simulink model "L4_MABX"  (R2018a)
settings: Solver=FixedStepDiscrete  StartTime=0.0  StopTime=Inf  FixedStep=0.01  RelTol=1e-3  EnableMultiTasking=on
PostLoadFcn:
  | , if any(exist('dsrtsu_mdlpostloadfcn', 'file') == [2, 3, 6]), try dsrtsu_mdlpostloadfcn('Execute', bdroot); catch fprintf('Error in PostLoadFcn (dsrtsu_mdlpostloadfcn) for model "%s":\n %s\n', bdroot, lasterr); end, end,
InitFcn:
  | disp([ptc_matlab_lib.isodatetime ' - ' bdroot(gcs) ' - Setting FixedStep to GLB_FIXED_STEP_SIZE_CPV']);
  | set_param(bdroot(gcs), 'FixedStep', num2str(GLB_FIXED_STEP_SIZE_CPV.Value));
undefined symbols (not defined in the file or in its folder): dsa_RTMapsManager, ENUM_CAN_STATUS_DIAG_T
libraries: PTC_MBDS_LIB x14, rtican x12, dsa_tcpip_lib x2, SUB_ECU_L4_MABX_HW_Interface_PIC_KW x2, rtiethxcplib x2, SUB_ECU_L4_MABX x1, simulink x1, rtmapslib x1
(part 1 of 2)
settings Model: DSRTSU_INTERNAL_RTI_VER=520  DSRTSU_INTERNAL_RTI_TYPE=rti1401  DSRTSU_INTERNAL_RTIFPGA=110  RTICANMMDATA=struct('GeneralSetupData',struct('modelroot','C:\Users\Gavin.Coelho\Repos\mabx\src','generalsettings',struct('filesettings',struct('destfolder',struct('Name','RTICANMM_FILES','Check',1),'buildfolder',struct('Name','.','Check',1),'AbsDestfolder',struct('Name','C:\Users\Gavin.Coelho\Repos\mabx\src\RTICANMM_FILES'),'AbsBuildfolder',struct('Name','C:\Users\Gavin.Coelho\Repos\mabx\src'))),'options',struct('addpaths',1,'rmpaths',1,'addtrcexclusion',logical(1),'cannavigator',struct('checkmonitoring',0),'show_usrtrc',0,'use_usrtrc',0),'advanced',struct('options',[1 1 1 1 1 1 1 1 1 1 1 1 1 1 1 1 1 1 1 1 1 1 1 1 1 1 1 1 1 1 1 1 1 1 1 1 1 1 1 1 1 1 1 1 1 1 1 1 1 1 1 1 1 1 1 1 1 1 1 1 1 1 1 1 1 1 1 1 1 1 1 1 1 1 1 1 1 1 1 1 1 1 1 1 1 1 1 1 1 1 1 1 1 1 1 1 1 1 1 1]),'MPSetup',{{}},'modelname','L4_MABX','block','L4_MABX'))  DSRTSU_INTERNAL_RTIFLEXRAYCONFIG=110  Creator=charles.swart  LastModifiedBy=Gavin.Coelho
settings SolverCC: AutoInsertRateTranBlk=on  InsertRTBMode=Always
settings DataIOCC: LimitDataPoints=on  SaveFormat=Array
settings OptimizationCC: BlockReduction=off  OptimizeBlockIOStorage=off  BufferReuse=off  GlobalBufferReuse=off  ExpressionFolding=off  LocalBlockOutputs=off  LifeSpan=inf  OptimizeDataStoreBuffers=off  BusAssignmentInplaceUpdate=off
settings DebuggingCC: SolverPrmCheckMsg=warning  MultiTaskDSMMsg=warning  MultiTaskCondExecSysMsg=warning  MultiTaskRateTransMsg=warning  ParameterPrecisionLossMsg=none  SignalLabelMismatchMsg=warning  UnconnectedInputMsg=error  UnconnectedLineMsg=error  StrictBusMsg=WarnOnBusTreatedAsVector  NonBusSignalsTreatedAsBus=warning  SFUnexpectedBacktrackingDiag=warning  SFNoUnconditionalDefaultTransitionDiag=warning  SFExecutionAtInitializationDiag=none
settings HardwareCC: ProdBitPerPointer=32  ProdBitPerSizeT=32  ProdBitPerPtrDiffT=32  ProdLargestAtomicInteger=Integer  ProdEndianess=BigEndian  ProdWordSize=32  ProdHWDeviceType=Custom Processor->Custom  TargetIntDivRoundTo=Zero  TargetEndianess=BigEndian  TargetHWDeviceType=Custom Processor->Custom
settings ModelReferenceCC: PropagateSignalLabelsOutOfModel=off
settings SFSimCC: MATLABDynamicMemAlloc=off
settings RTWCC: SystemTargetFile=rti1401.tlc  MakeCommand=make_rti  TemplateMakefile=rti1401.tmf  Description=dSPACE DS1401 Hardware Platform  GenerateReport=on
settings CodeAppCC: StateflowObjectComments=on
settings STFCustomTargetCC: ParMdlRefBuildCompliant=on  GRTInterface=off  SystemTargetFile=rti1401.tlc
settings GRTTargetCC: TargetLangStandard=C89/C90 (ANSI)  CompOptLevelCompliant=off  ConcurrentExecutionCompliant=off  CombineOutputUpdateFcns=off  MatFileLogging=off  CPPClassGenCompliant=off  UseToolchainInfoCompliant=off  ExtModeMexFile=noextcomm
settings ConfigComp: CovMetricSettings=dw  CovHtmlReporting=on  CovSaveCumulativeToWorkspaceVar=on  CovSaveSingleToWorkspaceVar=on  CovExternalEMLEnable=off  CovSFcnEnable=off

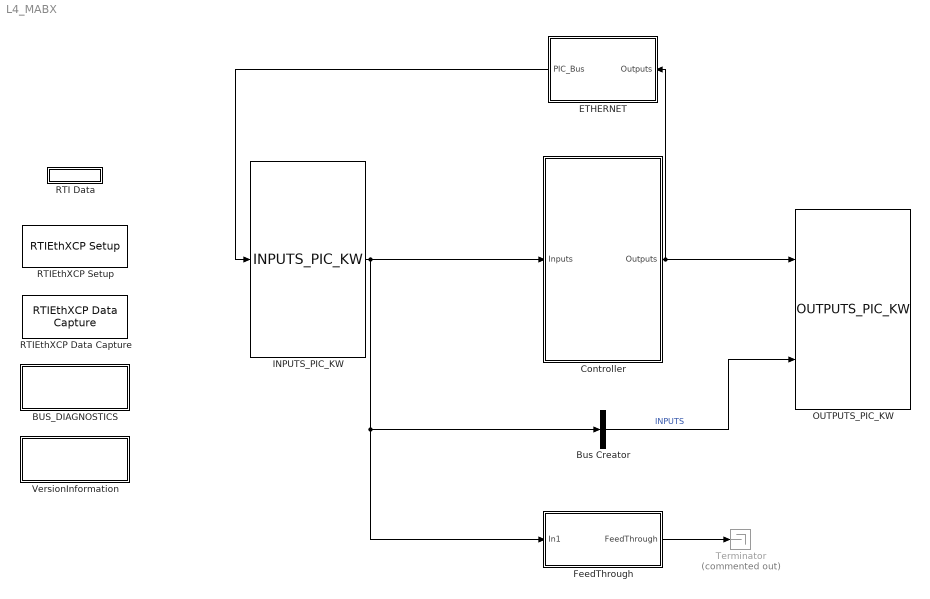
== system L4_MABX ==
  BUS_DIAGNOSTICS : Subsystem
  Bus Creator : BusCreator  Inputs=1
  Controller : Subsystem
  ETHERNET : Subsystem  AncestorBlock=SUB_ECU_L4_MABX_HW_Interface_PIC_KW/ETHERNET
  FeedThrough : Subsystem
  INPUTS_PIC_KW : SUB_ECU_L4_MABX_HW_Interface_PIC_KW/INPUTS_PIC_KW
      link override DIGITAL/Constant2: Value=1000
  OUTPUTS_PIC_KW : SUB_ECU_L4_MABX_HW_Interface_PIC_KW/OUTPUTS_PIC_KW
  RTI Data : Subsystem  Tag=struct('RTIDataServer',struct('RTIDataServerVs','2','RTIModelDescription','struct(''main'',''L4_MABX'',''sub'','''',''isMp'',0)'))  LoadFcn="if exist('rtidc'), try,  rtidc('DataHostBlockClbLoad', gcbh); catch, disp(['Warning: ''LoadFcn'' for RTI Data block failed: ' lasterr]); end, end,"  mask(RTI_DATA_HOST){}
      mask help:
      | RTI Data Block.
      | This block is used by RTI to store internal model-dependent data.
      | Please keep this block on the root level of the model. Deleting this block will result in data loss.
      |
      | NEVER DELETE OR COPY THIS BLOCK!
      settings: CopyFcn="if exist('rtidc'), try,  rtidc('DataHostBlockClbCopy', gcbh); catch, disp(['Warning: ''CopyFcn'' for RTI Data block failed: ' lasterr]); end, end,"  DeleteFcn="if exist('rtidc'), try,  rtidc('DataHostBlockClbDelete', gcbh); catch, disp(['Warning: ''DeleteFcn'' for RTI Data block failed: ' lasterr]); end, end,"  ModelCloseFcn="if exist('rtidc'), try,  rtidc('DataHostBlockClbModelClose', gcbh); catch, disp(['Warning: ''ModelCloseFcn'' for RTI Data block failed: ' lasterr]); end, end,"  PreSaveFcn="if exist('rtidc'), try,  rtidc('DataHostBlockClbPreSave', gcbh); catch, disp(['Warning: ''PreSaveFcn'' for RTI Data block failed: ' lasterr]); end, end,"  PostSaveFcn="if exist('rtidc'), try,  rtidc('DataHostBlockClbPostSave', gcbh); catch, disp(['Warning: ''PostSaveFcn'' for RTI Data block failed: ' lasterr]); end, end,"  NameChangeFcn="if exist('rtidc'), try,  rtidc('DataHostBlockClbNameChange', gcbh); catch, disp(['Warning: ''NameChangeFcn'' for RTI Data block failed: ' lasterr]); end, end,"
      mask Help:
      | RTI Data Block.
      | This block is used by RTI to store internal model-dependent data.
      | Please keep this block on the root level of the model. Deleting this block will result in data loss.
      | 
      | NEVER DELETE OR COPY THIS BLOCK!
      mask Display:
      | text(0.5, 0.5, 'RTI Data', 'HorizontalAlignment', 'center');
      | plot([1 0]);
  RTIEthXCP Data Capture : rtiethxcplib/RTIEthXCP Data Capture  Reserved1=[]  Reserved2=[]  Reserved3=[]  Reserved4=[]  DSProperties=struct('RTI',struct('Version',uint32(1),'BlockType',struct('isSLSource',uint8(0),'isSLSink',uint8(0),'isHWSource',uint8(0),'isHWSink',uint8(0),'isSetup',uint8(0),'isInline',uint8(1),'isNonInline',uint8(0),'isInterrupt',uint8(0),'isChannelwise',uint8(0)),'IOBoardType','RTIETHXCP','UnitType','NON_MESSAGE','Identifier','DATACAPTURE','DialogType','ML','BlockSet','RTIETHXCP','SlaveProcessor','NONE'))  RTIBlockInterface=struct('DialogFcn','guiethxcpdatacapture','BlockDisplay',{{['XCP Service #0\n<event channel name>\nCapture at task: <end>'],'center'}},'OutputPortsWidth',int32(0),'OutputPortsActive',0,'IconTransparency','on','InitLevel',3,'SampleTime',{{-1}},'BlockName',struct('Token',{{['RTIEthXCP Data Capture']}}))  RTIBlockParameters=struct('EventChannelName',{{'event_channel','OFF',[]}},'EventChannelNumber',{{0,'OFF',[]}},'DataCaptureAtEnd',{{1,'OFF',[0 1]}},'NumFormat',{{'dec','OFF',[]}},'SampleTime',{{-1,'OFF',[]}},'blockParam',{{0,'OFF',[]}},'TLCFileName',{{'rtiethxcpdatacapture','OFF',[]}})  RTISFcnParameters=struct('blockParam','struct','TLCFileName','char')  RTIBlockParaDefault=struct('EventChannelName','event_channel','EventChannelNumber',0,'DataCaptureAtEnd',1,'NumFormat','dec','SampleTime',-1,'blockParam',0,'TLCFileName','rtiethxcpdatacapture')
      settings: SourceProductName=dSPACE RTI XCP on Ethernet Blockset
  RTIEthXCP Setup : rtiethxcplib/RTIEthXCP Setup  Reserved1=[]  Reserved2=[]  Reserved3=[]  Reserved4=[]  DSProperties=struct('RTI',struct('Version',uint32(1),'BlockType',struct('isSLSource',uint8(0),'isSLSink',uint8(0),'isHWSource',uint8(0),'isHWSink',uint8(0),'isSetup',uint8(0),'isInline',uint8(1),'isNonInline',uint8(0),'isInterrupt',uint8(0),'isChannelwise',uint8(0)),'IOBoardType','RTIETHXCP','UnitType','NON_MESSAGE','Identifier','SETUP','DialogType','ML','BlockSet','RTIETHXCP','SlaveProcessor','NONE'))  RTIBlockInterface=struct('DialogFcn','guiethxcpsetup','BlockDisplay',{{['RTI Ethernet XCP\nSETUP'],'center'}},'OutputPortsWidth',int32(0),'OutputPortsActive',0,'IconTransparency','on','InitLevel',3,'SampleTime',{{-1}},'BlockName',struct('Token',{{['RTIEthXCP Setup']}}))  RTIBlockParameters=struct('BoardNo',{{1,'ON',[1 16]}},'UseStaticDAQLists',{{0,'OFF',[0 1]}},'Port',{{1234,'ON',[1 65535]}},'EthernetInterface',{{1,'OFF',[0 1]}},'blockParam',{{0,'OFF',[]}},'TLCFileName',{{'rtiethxcpsetup','OFF',[]}},'Address',{{'192.168.140.1','OFF',[]}},'VECUStruct',{{struct('EnableVECUA2LMerging',0,'SrcA2LFileName','','EVENTs',[]),'OFF',[]}})  RTISFcnParameters=struct('blockParam','struct','TLCFileName','char')  RTIBlockParaDefault=struct('BoardNo',1,'UseStaticDAQLists',0,'Port',1234,'EthernetInterface',0,'blockParam',0,'TLCFileName','rtiethxcpsetup','Address','127.0.0.1','VECUStruct',struct('EnableVECUA2LMerging',0,'SrcA2LFileName','','EVENTs',[]))
      settings: SourceProductName=dSPACE RTI XCP on Ethernet Blockset
  Terminator : Terminator  Commented=on
      settings: InitFcn=|
      | try
      |    MBDS_BlockCallback('Update', gcb);
      | end
  VersionInformation : Subsystem
  wires:
  FeedThrough/1(FeedThrough) -> Terminator/1
  INPUTS_PIC_KW/1 -> Bus Creator/1, FeedThrough/1(In1), Controller/1(Inputs)
  Controller/1(Outputs) -> OUTPUTS_PIC_KW/1, ETHERNET/1(Outputs)
  Bus Creator/1 -> OUTPUTS_PIC_KW/2  "INPUTS"
  ETHERNET/1(PIC_Bus) -> INPUTS_PIC_KW/1

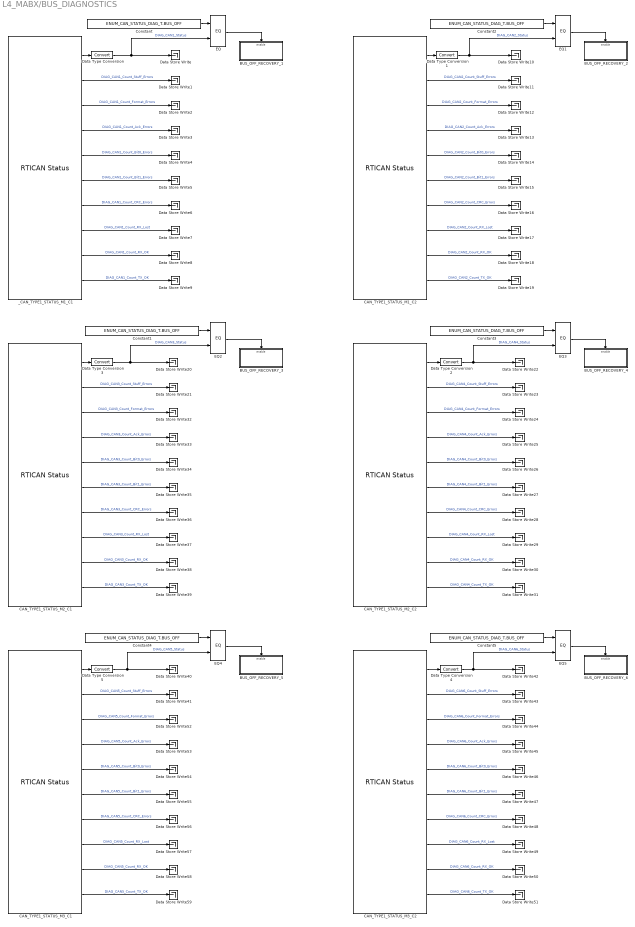
== system L4_MABX/BUS_DIAGNOSTICS ==
  BUS_OFF_RECOVERY_1 : Subsystem
  BUS_OFF_RECOVERY_2 : Subsystem
  BUS_OFF_RECOVERY_3 : Subsystem
  BUS_OFF_RECOVERY_4 : Subsystem
  BUS_OFF_RECOVERY_5 : Subsystem
  BUS_OFF_RECOVERY_6 : Subsystem
  CAN_TYPE1_STATUS_M1_C2 : rtican/RTICAN Status   Reserved1=[]  Reserved2=[]  Reserved3=[]  Reserved4=[]  DialogFcn=[]  UnitName=[]  SFcnRTICANStatus=[]  BoardTypeNo=[]  BoardNo=[]  ChannelNo=[]  Parameters=[]  Revision=[]  UnitValues=[]  DSProperties=struct('RTI',struct('Version',uint32(4),'BlockType',struct('isSLSource',uint8(1),'isSLSink',uint8(0),'isHWSource',uint8(0),'isHWSink',uint8(0),'isSetup',uint8(0),'isInline',uint8(1),'isNonInline',uint8(0),'isInterrupt',uint8(0),'isChannelwise',uint8(0)),'IOBoardType','RTICAN','UnitType','NON_MESSAGE','Identifier','STATUS','DialogType','ML','BlockSet','RTICAN','SlaveProcessor','CAN'))  RTIBlockInterface=struct('OutputPortsWidth',int32([1 1 1 1 1 1 1 1 1 1 1 1]),'OutputPortsActive',[1 1 1 1 1 1 1 1 1 1 0 0],'OutputPortsName',{{'Status',['Stuff errors'],['Format errors'],['Ack errors'],['Bit 0 errors'],['Bit 1 errors'],['CRC errors'],['RX lost'],['RX ok'],['TX ok'],['FT Status'],['FT error count']}},'OutputPortsDataType',{{'SS_UINT32','SS_UINT32','SS_UINT32','SS_UINT32','SS_UINT32','SS_UINT32','SS_UINT32','SS_UINT32','SS_UINT32','SS_UINT32','SS_UINT32','SS_UINT32'}},'DialogFcn','rtican_status_gui','BlockDisplay',{{'','center'}},'IconTransparency','on','ParameterTunableNames',{{}},'InitLevel',3,'BlockName',struct('Token',{{'CAN_TYPE','_STATUS_M','_C'}},'BlockParam',{{'BoardTypeNo','BoardNo','ChannelNo'}}),'SampleTime',{{2^-1}})  RTIBlockParameters=struct('BoardTypeNo',{{1,'OFF',[]}},'BoardNo',{{1,'ON',[1 16]}},'ChannelNo',{{2,'ON',[1 2]}},'Parameters',{{struct('general',struct('isFromLib',0,'StatusFlags',{{1;1;1;1;1;1;1;1;1;1;0;0}}),'options',struct('SampleTime',2^-1)),'OFF',[]}},'GroupId',{{struct('Group','RTICAN','No',2,'Behavior','NAMECHANGE','BlockType','SINK','NameChangeFlag',0),'OFF',[]}},'SFcnRTICANStatus',{{struct('Output',struct('Name',{'Status','StuffErrors','FormatErrors','AckErrors','Bit0Errors','Bit1Errors','CRCErrors','RXLost','RXOK','TXOK','FTStatus','FTErrorCount'},'Selected',{'yes','yes','yes','yes','yes','yes','yes','yes','yes','yes','no','no'}),'ControllerNo',2,'BoardNo',1,'BoardType','DS1','PortDatatype','UInt32'),'OFF',[]}},'TLCFileName',{{'rtican_status','OFF',[]}})  RTISFcnParameters=struct('SFcnRTICANStatus','struct','TLCFileName','char')  RTIBlockParaDefault=struct('BoardTypeNo',4302,'BoardNo',1,'ChannelNo',1,'Parameters',struct('general',struct('StatusFlags',{{1;1;1;1;1;1;1;1;1;1;0;0}},'isFromLib',1),'options',struct('SampleTime',2^-1)),'GroupId',struct('Group',{{'RTICAN'}},'No',1,'Behavior',{{'NAMECHANGE'}},'BlockType',{{'SINK'}},'NameChangeFlag',0),'SFcnRTICANStatus',struct('Output',struct('Name',{'Status','StuffErrors','FormatErrors','AckErrors','Bit0Errors','Bit1Errors','CRCErrors','RXLost','RXOK','TXOK','FTStatus','FTErrorCount'},'Selected',{'yes','yes','yes','yes','yes','yes','yes','yes','yes','yes','no','no'}),'ControllerNo',1,'BoardNo',1,'BoardType','DS4302','PortDatatype','real_T'),'TLCFileName','rtican_status')
      settings: AttributesFormatString=Group Id: RTICAN2\n  SourceProductName=dSPACE RTI CAN Blockset
  CAN_TYPE1_STATUS_M2_C1 : rtican/RTICAN Status   Reserved1=[]  Reserved2=[]  Reserved3=[]  Reserved4=[]  DialogFcn=[]  UnitName=[]  SFcnRTICANStatus=[]  BoardTypeNo=[]  BoardNo=[]  ChannelNo=[]  Parameters=[]  Revision=[]  UnitValues=[]  DSProperties=struct('RTI',struct('Version',uint32(4),'BlockType',struct('isSLSource',uint8(1),'isSLSink',uint8(0),'isHWSource',uint8(0),'isHWSink',uint8(0),'isSetup',uint8(0),'isInline',uint8(1),'isNonInline',uint8(0),'isInterrupt',uint8(0),'isChannelwise',uint8(0)),'IOBoardType','RTICAN','UnitType','NON_MESSAGE','Identifier','STATUS','DialogType','ML','BlockSet','RTICAN','SlaveProcessor','CAN'))  RTIBlockInterface=struct('OutputPortsWidth',int32([1 1 1 1 1 1 1 1 1 1 1 1]),'OutputPortsActive',[1 1 1 1 1 1 1 1 1 1 0 0],'OutputPortsName',{{'Status',['Stuff errors'],['Format errors'],['Ack errors'],['Bit 0 errors'],['Bit 1 errors'],['CRC errors'],['RX lost'],['RX ok'],['TX ok'],['FT Status'],['FT error count']}},'OutputPortsDataType',{{'SS_UINT32','SS_UINT32','SS_UINT32','SS_UINT32','SS_UINT32','SS_UINT32','SS_UINT32','SS_UINT32','SS_UINT32','SS_UINT32','SS_UINT32','SS_UINT32'}},'DialogFcn','rtican_status_gui','BlockDisplay',{{'','center'}},'IconTransparency','on','ParameterTunableNames',{{}},'InitLevel',3,'BlockName',struct('Token',{{'CAN_TYPE','_STATUS_M','_C'}},'BlockParam',{{'BoardTypeNo','BoardNo','ChannelNo'}}),'SampleTime',{{2^-1}})  RTIBlockParameters=struct('BoardTypeNo',{{1,'OFF',[]}},'BoardNo',{{2,'ON',[1 16]}},'ChannelNo',{{1,'ON',[1 2]}},'Parameters',{{struct('general',struct('isFromLib',0,'StatusFlags',{{1;1;1;1;1;1;1;1;1;1;0;0}}),'options',struct('SampleTime',2^-1)),'OFF',[]}},'GroupId',{{struct('Group','RTICAN','No',3,'Behavior','NAMECHANGE','BlockType','SINK','NameChangeFlag',0),'OFF',[]}},'SFcnRTICANStatus',{{struct('Output',struct('Name',{'Status','StuffErrors','FormatErrors','AckErrors','Bit0Errors','Bit1Errors','CRCErrors','RXLost','RXOK','TXOK','FTStatus','FTErrorCount'},'Selected',{'yes','yes','yes','yes','yes','yes','yes','yes','yes','yes','no','no'}),'ControllerNo',1,'BoardNo',2,'BoardType','DS1','PortDatatype','UInt32'),'OFF',[]}},'TLCFileName',{{'rtican_status','OFF',[]}})  RTISFcnParameters=struct('SFcnRTICANStatus','struct','TLCFileName','char')  RTIBlockParaDefault=struct('BoardTypeNo',4302,'BoardNo',1,'ChannelNo',1,'Parameters',struct('general',struct('StatusFlags',{{1;1;1;1;1;1;1;1;1;1;0;0}},'isFromLib',1),'options',struct('SampleTime',2^-1)),'GroupId',struct('Group',{{'RTICAN'}},'No',1,'Behavior',{{'NAMECHANGE'}},'BlockType',{{'SINK'}},'NameChangeFlag',0),'SFcnRTICANStatus',struct('Output',struct('Name',{'Status','StuffErrors','FormatErrors','AckErrors','Bit0Errors','Bit1Errors','CRCErrors','RXLost','RXOK','TXOK','FTStatus','FTErrorCount'},'Selected',{'yes','yes','yes','yes','yes','yes','yes','yes','yes','yes','no','no'}),'ControllerNo',1,'BoardNo',1,'BoardType','DS4302','PortDatatype','real_T'),'TLCFileName','rtican_status')
      settings: AttributesFormatString=Group Id: RTICAN3\n  SourceProductName=dSPACE RTI CAN Blockset
  CAN_TYPE1_STATUS_M2_C2 : rtican/RTICAN Status   Reserved1=[]  Reserved2=[]  Reserved3=[]  Reserved4=[]  DialogFcn=[]  UnitName=[]  SFcnRTICANStatus=[]  BoardTypeNo=[]  BoardNo=[]  ChannelNo=[]  Parameters=[]  Revision=[]  UnitValues=[]  DSProperties=struct('RTI',struct('Version',uint32(4),'BlockType',struct('isSLSource',uint8(1),'isSLSink',uint8(0),'isHWSource',uint8(0),'isHWSink',uint8(0),'isSetup',uint8(0),'isInline',uint8(1),'isNonInline',uint8(0),'isInterrupt',uint8(0),'isChannelwise',uint8(0)),'IOBoardType','RTICAN','UnitType','NON_MESSAGE','Identifier','STATUS','DialogType','ML','BlockSet','RTICAN','SlaveProcessor','CAN'))  RTIBlockInterface=struct('OutputPortsWidth',int32([1 1 1 1 1 1 1 1 1 1 1 1]),'OutputPortsActive',[1 1 1 1 1 1 1 1 1 1 0 0],'OutputPortsName',{{'Status',['Stuff errors'],['Format errors'],['Ack errors'],['Bit 0 errors'],['Bit 1 errors'],['CRC errors'],['RX lost'],['RX ok'],['TX ok'],['FT Status'],['FT error count']}},'OutputPortsDataType',{{'SS_UINT32','SS_UINT32','SS_UINT32','SS_UINT32','SS_UINT32','SS_UINT32','SS_UINT32','SS_UINT32','SS_UINT32','SS_UINT32','SS_UINT32','SS_UINT32'}},'DialogFcn','rtican_status_gui','BlockDisplay',{{'','center'}},'IconTransparency','on','ParameterTunableNames',{{}},'InitLevel',3,'BlockName',struct('Token',{{'CAN_TYPE','_STATUS_M','_C'}},'BlockParam',{{'BoardTypeNo','BoardNo','ChannelNo'}}),'SampleTime',{{2^-1}})  RTIBlockParameters=struct('BoardTypeNo',{{1,'OFF',[]}},'BoardNo',{{2,'ON',[1 16]}},'ChannelNo',{{2,'ON',[1 2]}},'Parameters',{{struct('general',struct('isFromLib',0,'StatusFlags',{{1;1;1;1;1;1;1;1;1;1;0;0}}),'options',struct('SampleTime',2^-1)),'OFF',[]}},'GroupId',{{struct('Group','RTICAN','No',4,'Behavior','NAMECHANGE','BlockType','SINK','NameChangeFlag',0),'OFF',[]}},'SFcnRTICANStatus',{{struct('Output',struct('Name',{'Status','StuffErrors','FormatErrors','AckErrors','Bit0Errors','Bit1Errors','CRCErrors','RXLost','RXOK','TXOK','FTStatus','FTErrorCount'},'Selected',{'yes','yes','yes','yes','yes','yes','yes','yes','yes','yes','no','no'}),'ControllerNo',2,'BoardNo',2,'BoardType','DS1','PortDatatype','UInt32'),'OFF',[]}},'TLCFileName',{{'rtican_status','OFF',[]}})  RTISFcnParameters=struct('SFcnRTICANStatus','struct','TLCFileName','char')  RTIBlockParaDefault=struct('BoardTypeNo',4302,'BoardNo',1,'ChannelNo',1,'Parameters',struct('general',struct('StatusFlags',{{1;1;1;1;1;1;1;1;1;1;0;0}},'isFromLib',1),'options',struct('SampleTime',2^-1)),'GroupId',struct('Group',{{'RTICAN'}},'No',1,'Behavior',{{'NAMECHANGE'}},'BlockType',{{'SINK'}},'NameChangeFlag',0),'SFcnRTICANStatus',struct('Output',struct('Name',{'Status','StuffErrors','FormatErrors','AckErrors','Bit0Errors','Bit1Errors','CRCErrors','RXLost','RXOK','TXOK','FTStatus','FTErrorCount'},'Selected',{'yes','yes','yes','yes','yes','yes','yes','yes','yes','yes','no','no'}),'ControllerNo',1,'BoardNo',1,'BoardType','DS4302','PortDatatype','real_T'),'TLCFileName','rtican_status')
      settings: AttributesFormatString=Group Id: RTICAN4\n  SourceProductName=dSPACE RTI CAN Blockset
  CAN_TYPE1_STATUS_M3_C1 : rtican/RTICAN Status   Reserved1=[]  Reserved2=[]  Reserved3=[]  Reserved4=[]  DialogFcn=[]  UnitName=[]  SFcnRTICANStatus=[]  BoardTypeNo=[]  BoardNo=[]  ChannelNo=[]  Parameters=[]  Revision=[]  UnitValues=[]  DSProperties=struct('RTI',struct('Version',uint32(4),'BlockType',struct('isSLSource',uint8(1),'isSLSink',uint8(0),'isHWSource',uint8(0),'isHWSink',uint8(0),'isSetup',uint8(0),'isInline',uint8(1),'isNonInline',uint8(0),'isInterrupt',uint8(0),'isChannelwise',uint8(0)),'IOBoardType','RTICAN','UnitType','NON_MESSAGE','Identifier','STATUS','DialogType','ML','BlockSet','RTICAN','SlaveProcessor','CAN'))  RTIBlockInterface=struct('OutputPortsWidth',int32([1 1 1 1 1 1 1 1 1 1 1 1]),'OutputPortsActive',[1 1 1 1 1 1 1 1 1 1 0 0],'OutputPortsName',{{'Status',['Stuff errors'],['Format errors'],['Ack errors'],['Bit 0 errors'],['Bit 1 errors'],['CRC errors'],['RX lost'],['RX ok'],['TX ok'],['FT Status'],['FT error count']}},'OutputPortsDataType',{{'SS_UINT32','SS_UINT32','SS_UINT32','SS_UINT32','SS_UINT32','SS_UINT32','SS_UINT32','SS_UINT32','SS_UINT32','SS_UINT32','SS_UINT32','SS_UINT32'}},'DialogFcn','rtican_status_gui','BlockDisplay',{{'','center'}},'IconTransparency','on','ParameterTunableNames',{{}},'InitLevel',3,'BlockName',struct('Token',{{'CAN_TYPE','_STATUS_M','_C'}},'BlockParam',{{'BoardTypeNo','BoardNo','ChannelNo'}}),'SampleTime',{{2^-1}})  RTIBlockParameters=struct('BoardTypeNo',{{1,'OFF',[]}},'BoardNo',{{3,'ON',[1 16]}},'ChannelNo',{{1,'ON',[1 2]}},'Parameters',{{struct('general',struct('isFromLib',0,'StatusFlags',{{1;1;1;1;1;1;1;1;1;1;0;0}}),'options',struct('SampleTime',2^-1)),'OFF',[]}},'GroupId',{{struct('Group','RTICAN','No',5,'Behavior','NAMECHANGE','BlockType','SINK','NameChangeFlag',0),'OFF',[]}},'SFcnRTICANStatus',{{struct('Output',struct('Name',{'Status','StuffErrors','FormatErrors','AckErrors','Bit0Errors','Bit1Errors','CRCErrors','RXLost','RXOK','TXOK','FTStatus','FTErrorCount'},'Selected',{'yes','yes','yes','yes','yes','yes','yes','yes','yes','yes','no','no'}),'ControllerNo',1,'BoardNo',3,'BoardType','DS1','PortDatatype','UInt32'),'OFF',[]}},'TLCFileName',{{'rtican_status','OFF',[]}})  RTISFcnParameters=struct('SFcnRTICANStatus','struct','TLCFileName','char')  RTIBlockParaDefault=struct('BoardTypeNo',4302,'BoardNo',1,'ChannelNo',1,'Parameters',struct('general',struct('StatusFlags',{{1;1;1;1;1;1;1;1;1;1;0;0}},'isFromLib',1),'options',struct('SampleTime',2^-1)),'GroupId',struct('Group',{{'RTICAN'}},'No',1,'Behavior',{{'NAMECHANGE'}},'BlockType',{{'SINK'}},'NameChangeFlag',0),'SFcnRTICANStatus',struct('Output',struct('Name',{'Status','StuffErrors','FormatErrors','AckErrors','Bit0Errors','Bit1Errors','CRCErrors','RXLost','RXOK','TXOK','FTStatus','FTErrorCount'},'Selected',{'yes','yes','yes','yes','yes','yes','yes','yes','yes','yes','no','no'}),'ControllerNo',1,'BoardNo',1,'BoardType','DS4302','PortDatatype','real_T'),'TLCFileName','rtican_status')
      settings: AttributesFormatString=Group Id: RTICAN5\n  SourceProductName=dSPACE RTI CAN Blockset
  CAN_TYPE1_STATUS_M3_C2 : rtican/RTICAN Status   Reserved1=[]  Reserved2=[]  Reserved3=[]  Reserved4=[]  DialogFcn=[]  UnitName=[]  SFcnRTICANStatus=[]  BoardTypeNo=[]  BoardNo=[]  ChannelNo=[]  Parameters=[]  Revision=[]  UnitValues=[]  DSProperties=struct('RTI',struct('Version',uint32(4),'BlockType',struct('isSLSource',uint8(1),'isSLSink',uint8(0),'isHWSource',uint8(0),'isHWSink',uint8(0),'isSetup',uint8(0),'isInline',uint8(1),'isNonInline',uint8(0),'isInterrupt',uint8(0),'isChannelwise',uint8(0)),'IOBoardType','RTICAN','UnitType','NON_MESSAGE','Identifier','STATUS','DialogType','ML','BlockSet','RTICAN','SlaveProcessor','CAN'))  RTIBlockInterface=struct('OutputPortsWidth',int32([1 1 1 1 1 1 1 1 1 1 1 1]),'OutputPortsActive',[1 1 1 1 1 1 1 1 1 1 0 0],'OutputPortsName',{{'Status',['Stuff errors'],['Format errors'],['Ack errors'],['Bit 0 errors'],['Bit 1 errors'],['CRC errors'],['RX lost'],['RX ok'],['TX ok'],['FT Status'],['FT error count']}},'OutputPortsDataType',{{'SS_UINT32','SS_UINT32','SS_UINT32','SS_UINT32','SS_UINT32','SS_UINT32','SS_UINT32','SS_UINT32','SS_UINT32','SS_UINT32','SS_UINT32','SS_UINT32'}},'DialogFcn','rtican_status_gui','BlockDisplay',{{'','center'}},'IconTransparency','on','ParameterTunableNames',{{}},'InitLevel',3,'BlockName',struct('Token',{{'CAN_TYPE','_STATUS_M','_C'}},'BlockParam',{{'BoardTypeNo','BoardNo','ChannelNo'}}),'SampleTime',{{2^-1}})  RTIBlockParameters=struct('BoardTypeNo',{{1,'OFF',[]}},'BoardNo',{{3,'ON',[1 16]}},'ChannelNo',{{2,'ON',[1 2]}},'Parameters',{{struct('general',struct('isFromLib',0,'StatusFlags',{{1;1;1;1;1;1;1;1;1;1;0;0}}),'options',struct('SampleTime',2^-1)),'OFF',[]}},'GroupId',{{struct('Group','RTICAN','No',6,'Behavior','NAMECHANGE','BlockType','SINK','NameChangeFlag',0),'OFF',[]}},'SFcnRTICANStatus',{{struct('Output',struct('Name',{'Status','StuffErrors','FormatErrors','AckErrors','Bit0Errors','Bit1Errors','CRCErrors','RXLost','RXOK','TXOK','FTStatus','FTErrorCount'},'Selected',{'yes','yes','yes','yes','yes','yes','yes','yes','yes','yes','no','no'}),'ControllerNo',2,'BoardNo',3,'BoardType','DS1','PortDatatype','UInt32'),'OFF',[]}},'TLCFileName',{{'rtican_status','OFF',[]}})  RTISFcnParameters=struct('SFcnRTICANStatus','struct','TLCFileName','char')  RTIBlockParaDefault=struct('BoardTypeNo',4302,'BoardNo',1,'ChannelNo',1,'Parameters',struct('general',struct('StatusFlags',{{1;1;1;1;1;1;1;1;1;1;0;0}},'isFromLib',1),'options',struct('SampleTime',2^-1)),'GroupId',struct('Group',{{'RTICAN'}},'No',1,'Behavior',{{'NAMECHANGE'}},'BlockType',{{'SINK'}},'NameChangeFlag',0),'SFcnRTICANStatus',struct('Output',struct('Name',{'Status','StuffErrors','FormatErrors','AckErrors','Bit0Errors','Bit1Errors','CRCErrors','RXLost','RXOK','TXOK','FTStatus','FTErrorCount'},'Selected',{'yes','yes','yes','yes','yes','yes','yes','yes','yes','yes','no','no'}),'ControllerNo',1,'BoardNo',1,'BoardType','DS4302','PortDatatype','real_T'),'TLCFileName','rtican_status')
      settings: AttributesFormatString=Group Id: RTICAN6\n  SourceProductName=dSPACE RTI CAN Blockset
  Constant{,1..5} (6 alike) : Constant  Value=ENUM_CAN_STATUS_DIAG_T.BUS_OFF
  Data Store Write{,1..59} (60 alike) : Terminator
      settings: InitFcn=|
      | try
      |    MBDS_BlockCallback('Update', gcb);
      | end
  Data Type Conversion{,1..5} (6 alike) : DataTypeConversion  SaturateOnIntegerOverflow=on
  EQ{,1..5} (6 alike) : PTC_MBDS_LIB/MBDS Standard Library/Basic Operations/Logic and Bit Operations/EQ  InputSameDT=on  PTC_MBDS_BlockVersion=5.41  PTC_BlockType=PTC_MBDS_EQ
      settings: SourceProductName=PACCAR Technical Center MBDS Library
  _CAN_TYPE1_STATUS_M1_C1 : rtican/RTICAN Status   Reserved1=[]  Reserved2=[]  Reserved3=[]  Reserved4=[]  DialogFcn=[]  UnitName=[]  SFcnRTICANStatus=[]  BoardTypeNo=[]  BoardNo=[]  ChannelNo=[]  Parameters=[]  Revision=[]  UnitValues=[]  DSProperties=struct('RTI',struct('Version',uint32(4),'BlockType',struct('isSLSource',uint8(1),'isSLSink',uint8(0),'isHWSource',uint8(0),'isHWSink',uint8(0),'isSetup',uint8(0),'isInline',uint8(1),'isNonInline',uint8(0),'isInterrupt',uint8(0),'isChannelwise',uint8(0)),'IOBoardType','RTICAN','UnitType','NON_MESSAGE','Identifier','STATUS','DialogType','ML','BlockSet','RTICAN','SlaveProcessor','CAN'))  RTIBlockInterface=struct('OutputPortsWidth',int32([1 1 1 1 1 1 1 1 1 1 1 1]),'OutputPortsActive',[1 1 1 1 1 1 1 1 1 1 0 0],'OutputPortsName',{{'Status',['Stuff errors'],['Format errors'],['Ack errors'],['Bit 0 errors'],['Bit 1 errors'],['CRC errors'],['RX lost'],['RX ok'],['TX ok'],['FT Status'],['FT error count']}},'OutputPortsDataType',{{'SS_UINT32','SS_UINT32','SS_UINT32','SS_UINT32','SS_UINT32','SS_UINT32','SS_UINT32','SS_UINT32','SS_UINT32','SS_UINT32','SS_UINT32','SS_UINT32'}},'DialogFcn','rtican_status_gui','BlockDisplay',{{'','center'}},'IconTransparency','on','ParameterTunableNames',{{}},'InitLevel',3,'BlockName',struct('Token',{{'CAN_TYPE','_STATUS_M','_C'}},'BlockParam',{{'BoardTypeNo','BoardNo','ChannelNo'}}),'SampleTime',{{2^-1}})  RTIBlockParameters=struct('BoardTypeNo',{{1,'OFF',[]}},'BoardNo',{{1,'ON',[1 16]}},'ChannelNo',{{1,'ON',[1 2]}},'Parameters',{{struct('general',struct('StatusFlags',{{1;1;1;1;1;1;1;1;1;1;0;0}},'isFromLib',0),'options',struct('SampleTime',2^-1)),'OFF',[]}},'GroupId',{{struct('Group','RTICAN','No',1,'Behavior','NAMECHANGE','BlockType','SINK','NameChangeFlag',0),'OFF',[]}},'SFcnRTICANStatus',{{struct('Output',struct('Name',{'Status','StuffErrors','FormatErrors','AckErrors','Bit0Errors','Bit1Errors','CRCErrors','RXLost','RXOK','TXOK','FTStatus','FTErrorCount'},'Selected',{'yes','yes','yes','yes','yes','yes','yes','yes','yes','yes','no','no'}),'ControllerNo',1,'BoardNo',1,'BoardType','DS1','PortDatatype','UInt32'),'OFF',[]}},'TLCFileName',{{'rtican_status','OFF',[]}})  RTISFcnParameters=struct('SFcnRTICANStatus','struct','TLCFileName','char')  RTIBlockParaDefault=struct('BoardTypeNo',4302,'BoardNo',1,'ChannelNo',1,'Parameters',struct('general',struct('StatusFlags',{{1;1;1;1;1;1;1;1;1;1;0;0}},'isFromLib',1),'options',struct('SampleTime',2^-1)),'GroupId',struct('Group',{{'RTICAN'}},'No',1,'Behavior',{{'NAMECHANGE'}},'BlockType',{{'SINK'}},'NameChangeFlag',0),'SFcnRTICANStatus',struct('Output',struct('Name',{'Status','StuffErrors','FormatErrors','AckErrors','Bit0Errors','Bit1Errors','CRCErrors','RXLost','RXOK','TXOK','FTStatus','FTErrorCount'},'Selected',{'yes','yes','yes','yes','yes','yes','yes','yes','yes','yes','no','no'}),'ControllerNo',1,'BoardNo',1,'BoardType','DS4302','PortDatatype','real_T'),'TLCFileName','rtican_status')
      settings: AttributesFormatString=Group Id: RTICAN1\n  SourceProductName=dSPACE RTI CAN Blockset
  wires:
  Constant/1 -> EQ/1
  _CAN_TYPE1_STATUS_M1_C1/1 -> Data Type Conversion/1
  EQ/1 -> BUS_OFF_RECOVERY_1/Enable
  _CAN_TYPE1_STATUS_M1_C1/2 -> Data Store Write1/1  "DIAG_CAN1_Count_Stuff_Errors"
  _CAN_TYPE1_STATUS_M1_C1/8 -> Data Store Write7/1  "DIAG_CAN1_Count_RX_Lost"
  _CAN_TYPE1_STATUS_M1_C1/7 -> Data Store Write6/1  "DIAG_CAN1_Count_CRC_Errors"
  _CAN_TYPE1_STATUS_M1_C1/6 -> Data Store Write5/1  "DIAG_CAN1_Count_Bit1_Errors"
  _CAN_TYPE1_STATUS_M1_C1/5 -> Data Store Write4/1  "DIAG_CAN1_Count_Bit0_Errors"
  _CAN_TYPE1_STATUS_M1_C1/4 -> Data Store Write3/1  "DIAG_CAN1_Count_Ack_Errors"
  _CAN_TYPE1_STATUS_M1_C1/3 -> Data Store Write2/1  "DIAG_CAN1_Count_Format_Errors"
  _CAN_TYPE1_STATUS_M1_C1/9 -> Data Store Write8/1  "DIAG_CAN1_Count_RX_OK"
  _CAN_TYPE1_STATUS_M1_C1/10 -> Data Store Write9/1  "DIAG_CAN1_Count_TX_OK"
  Constant2/1 -> EQ1/1
  CAN_TYPE1_STATUS_M1_C2/1 -> Data Type Conversion1/1
  EQ1/1 -> BUS_OFF_RECOVERY_2/Enable
  CAN_TYPE1_STATUS_M1_C2/2 -> Data Store Write11/1  "DIAG_CAN2_Count_Stuff_Errors"
  CAN_TYPE1_STATUS_M1_C2/8 -> Data Store Write17/1  "DIAG_CAN2_Count_RX_Lost"
  CAN_TYPE1_STATUS_M1_C2/7 -> Data Store Write16/1  "DIAG_CAN2_Count_CRC_Errors"
  CAN_TYPE1_STATUS_M1_C2/6 -> Data Store Write15/1  "DIAG_CAN2_Count_Bit1_Errors"
  CAN_TYPE1_STATUS_M1_C2/5 -> Data Store Write14/1  "DIAG_CAN2_Count_Bit0_Errors"
  CAN_TYPE1_STATUS_M1_C2/4 -> Data Store Write13/1  "DIAG_CAN2_Count_Ack_Errors"
  CAN_TYPE1_STATUS_M1_C2/3 -> Data Store Write12/1  "DIAG_CAN2_Count_Format_Errors"
  CAN_TYPE1_STATUS_M1_C2/9 -> Data Store Write18/1  "DIAG_CAN2_Count_RX_OK"
  CAN_TYPE1_STATUS_M1_C2/10 -> Data Store Write19/1  "DIAG_CAN2_Count_TX_OK"
  Constant1/1 -> EQ2/1
  CAN_TYPE1_STATUS_M2_C1/1 -> Data Type Conversion3/1
  EQ2/1 -> BUS_OFF_RECOVERY_3/Enable
  CAN_TYPE1_STATUS_M2_C1/2 -> Data Store Write21/1  "DIAG_CAN3_Count_Stuff_Errors"
  CAN_TYPE1_STATUS_M2_C1/8 -> Data Store Write37/1  "DIAG_CAN3_Count_RX_Lost"
  CAN_TYPE1_STATUS_M2_C1/7 -> Data Store Write36/1  "DIAG_CAN3_Count_CRC_Errors"
  CAN_TYPE1_STATUS_M2_C1/6 -> Data Store Write35/1  "DIAG_CAN3_Count_Bit1_Errors"
  CAN_TYPE1_STATUS_M2_C1/5 -> Data Store Write34/1  "DIAG_CAN3_Count_Bit0_Errors"
  CAN_TYPE1_STATUS_M2_C1/4 -> Data Store Write33/1  "DIAG_CAN3_Count_Ack_Errors"
  CAN_TYPE1_STATUS_M2_C1/3 -> Data Store Write32/1  "DIAG_CAN3_Count_Format_Errors"
  CAN_TYPE1_STATUS_M2_C1/9 -> Data Store Write38/1  "DIAG_CAN3_Count_RX_OK"
  CAN_TYPE1_STATUS_M2_C1/10 -> Data Store Write39/1  "DIAG_CAN3_Count_TX_OK"
  Constant3/1 -> EQ3/1
  CAN_TYPE1_STATUS_M2_C2/1 -> Data Type Conversion2/1
  EQ3/1 -> BUS_OFF_RECOVERY_4/Enable
  CAN_TYPE1_STATUS_M2_C2/2 -> Data Store Write23/1  "DIAG_CAN4_Count_Stuff_Errors"
  CAN_TYPE1_STATUS_M2_C2/8 -> Data Store Write29/1  "DIAG_CAN4_Count_RX_Lost"
  CAN_TYPE1_STATUS_M2_C2/7 -> Data Store Write28/1  "DIAG_CAN4_Count_CRC_Errors"
  CAN_TYPE1_STATUS_M2_C2/6 -> Data Store Write27/1  "DIAG_CAN4_Count_Bit1_Errors"
  CAN_TYPE1_STATUS_M2_C2/5 -> Data Store Write26/1  "DIAG_CAN4_Count_Bit0_Errors"
  CAN_TYPE1_STATUS_M2_C2/4 -> Data Store Write25/1  "DIAG_CAN4_Count_Ack_Errors"
  CAN_TYPE1_STATUS_M2_C2/3 -> Data Store Write24/1  "DIAG_CAN4_Count_Format_Errors"
  CAN_TYPE1_STATUS_M2_C2/9 -> Data Store Write30/1  "DIAG_CAN4_Count_RX_OK"
  CAN_TYPE1_STATUS_M2_C2/10 -> Data Store Write31/1  "DIAG_CAN4_Count_TX_OK"
  Constant4/1 -> EQ4/1
  CAN_TYPE1_STATUS_M3_C1/1 -> Data Type Conversion5/1
  EQ4/1 -> BUS_OFF_RECOVERY_5/Enable
  CAN_TYPE1_STATUS_M3_C1/2 -> Data Store Write41/1  "DIAG_CAN5_Count_Stuff_Errors"
  CAN_TYPE1_STATUS_M3_C1/8 -> Data Store Write57/1  "DIAG_CAN5_Count_RX_Lost"
  CAN_TYPE1_STATUS_M3_C1/7 -> Data Store Write56/1  "DIAG_CAN5_Count_CRC_Errors"
  CAN_TYPE1_STATUS_M3_C1/6 -> Data Store Write55/1  "DIAG_CAN5_Count_Bit1_Errors"
  CAN_TYPE1_STATUS_M3_C1/5 -> Data Store Write54/1  "DIAG_CAN5_Count_Bit0_Errors"
  CAN_TYPE1_STATUS_M3_C1/4 -> Data Store Write53/1  "DIAG_CAN5_Count_Ack_Errors"
  CAN_TYPE1_STATUS_M3_C1/3 -> Data Store Write52/1  "DIAG_CAN5_Count_Format_Errors"
  CAN_TYPE1_STATUS_M3_C1/9 -> Data Store Write58/1  "DIAG_CAN5_Count_RX_OK"
  CAN_TYPE1_STATUS_M3_C1/10 -> Data Store Write59/1  "DIAG_CAN5_Count_TX_OK"
  Constant5/1 -> EQ5/1
  CAN_TYPE1_STATUS_M3_C2/1 -> Data Type Conversion4/1
  EQ5/1 -> BUS_OFF_RECOVERY_6/Enable
  CAN_TYPE1_STATUS_M3_C2/2 -> Data Store Write43/1  "DIAG_CAN6_Count_Stuff_Errors"
  CAN_TYPE1_STATUS_M3_C2/8 -> Data Store Write49/1  "DIAG_CAN6_Count_RX_Lost"
  CAN_TYPE1_STATUS_M3_C2/7 -> Data Store Write48/1  "DIAG_CAN6_Count_CRC_Errors"
  CAN_TYPE1_STATUS_M3_C2/6 -> Data Store Write47/1  "DIAG_CAN6_Count_Bit1_Errors"
  CAN_TYPE1_STATUS_M3_C2/5 -> Data Store Write46/1  "DIAG_CAN6_Count_Bit0_Errors"
  CAN_TYPE1_STATUS_M3_C2/4 -> Data Store Write45/1  "DIAG_CAN6_Count_Ack_Errors"
  CAN_TYPE1_STATUS_M3_C2/3 -> Data Store Write44/1  "DIAG_CAN6_Count_Format_Errors"
  CAN_TYPE1_STATUS_M3_C2/9 -> Data Store Write50/1  "DIAG_CAN6_Count_RX_OK"
  CAN_TYPE1_STATUS_M3_C2/10 -> Data Store Write51/1  "DIAG_CAN6_Count_TX_OK"
  Data Type Conversion/1 -> EQ/2, Data Store Write/1  "DIAG_CAN1_Status"
  Data Type Conversion1/1 -> EQ1/2, Data Store Write10/1  "DIAG_CAN2_Status"
  Data Type Conversion2/1 -> EQ3/2, Data Store Write22/1  "DIAG_CAN4_Status"
  Data Type Conversion3/1 -> EQ2/2, Data Store Write20/1  "DIAG_CAN3_Status"
  Data Type Conversion4/1 -> EQ5/2, Data Store Write42/1  "DIAG_CAN6_Status"
  Data Type Conversion5/1 -> EQ4/2, Data Store Write40/1  "DIAG_CAN5_Status"

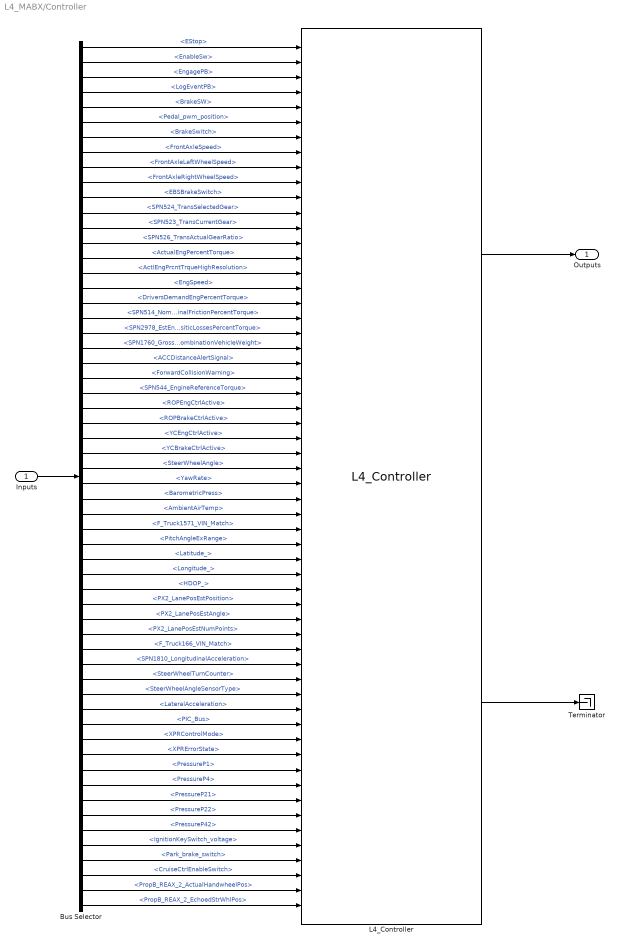
== system L4_MABX/Controller ==
  Inputs : Inport
  Bus Selector : BusSelector  OutputSignals=DIO_Bus.EStop,DIO_Bus.EnableSw,DIO_Bus.EngagePB,DIO_Bus.LogEventPB,DIO_Bus.BrakeSW,DIO_Bus.Pedal_pwm_position,CAN.CCVS1_31.CCVS31Data.BrakeSwitch,CAN.EBC2_0B.FrontAxleSpeed,CAN.HRW_0B.FrontAxleLeftWheelSpeed,CAN.HRW_0B.FrontAxleRightWheelSpeed,CAN.EBC1_8B.EBSBrakeSwitch,CAN.ETC2_03.SPN524_TransSelectedGear,CAN.ETC2_03.SPN523_TransCurrentGear,CAN.ETC2_03.SPN526_TransActualGearRatio,CAN.EEC1_00.ActualEngPercentTorque,CAN.EEC1_00.ActlEngPrcntTrqueHighResolution,CAN.EEC1_00.EngSpeed,CAN.EEC1_00.DriversDemandEngPercentTorque,CAN.EEC3_00.SPN514_NominalFrictionPercentTorque,CAN.EEC3_00.SPN2978_EstEngParasiticLossesPercentTorque,CAN.CVW_0B.SPN1760_GrossCombinationVehicleWeight,CAN.ACC1_2A.ACCDistanceAlertSignal,CAN.ACC1_2A.ForwardCollisionWarning,CAN.EC1_00.SPN544_EngineReferenceTorque,CAN.VDC1_0B.ROPEngCtrlActive,CAN.VDC1_0B.ROPBrakeCtrlActive,CAN.VDC1_0B.YCEngCtrlActive,CAN.VDC1_0B.YCBrakeCtrlActive,CAN.VDC2_0B.SteerWheelAngle,CAN.VDC2_0B.YawRate,CAN.AMB_00.AMB_00Data.BarometricPress,CAN.AMB_00.AMB_00Data.AmbientAirTemp,CAN.VI_00.Signals.F_Truck1571_VIN_Match,CAN.SSI2_03.PitchAngleExRange,CAN.PosRapidUpdate.Latitude_,CAN.PosRapidUpdate.Longitude_,CAN.GNSSDOPs.HDOP_,CAN.PX2_Lane.LanePosEst.PX2_LanePosEstPosition,CAN.PX2_Lane.LanePosEst.PX2_LanePosEstAngle,CAN.PX2_Lane.LanePosEst.PX2_LanePosEstNumPoints,CAN.VI_00.Signals.F_Truck166_VIN_Match,CAN.VDC2_0B.SPN1810_LongitudinalAcceleration,CAN.VDC2_0B.SteerWheelTurnCounter,CAN.VDC2_0B.SteerWheelAngleSensorType,CAN.VDC2_0B.LateralAcceleration,PIC_Bus,CAN.Prop2C2_Status_30.XPRControlMode,CAN.Prop2C2_Status_30.XPRErrorState,CAN.Prop2C2_Status_30.PressureP1,CAN.Prop2C2_Status_30.PressureP4,CAN.Prop2C2_Status_30.PressureP21,CAN.Prop2C2_Status_30.PressureP22,CAN.Prop2C2_Status_30.PressureP42,DIO_Bus.IgnitionKeySwitch_voltage,CAN.CCVS1_31.CCVS31Data.Park_brake_switch,CAN.CCVS1_31.CCVS31Data.CruiseCtrlEnableSwitch,CAN.PropN_REAX_2.PropB_REAX_2_ActualHandwheelPos,CAN.PropN_REAX_2.PropB_REAX_2_EchoedStrWhlPos
  L4_Controller : SUB_ECU_L4_MABX/L4_Controller
  Terminator : Terminator
      settings: InitFcn=|
      | try
      |    MBDS_BlockCallback('Update', gcb);
      | end
  Outputs : Outport
  wires:
  L4_Controller/1 -> Outputs/1
  L4_Controller/2 -> Terminator/1
  Inputs/1 -> Bus Selector/1
  Bus Selector/1 -> L4_Controller/1  "<EStop>"
  Bus Selector/6 -> L4_Controller/6  "<Pedal_pwm_position>"
  Bus Selector/7 -> L4_Controller/7  "<BrakeSwitch>"
  Bus Selector/8 -> L4_Controller/8  "<FrontAxleSpeed>"
  Bus Selector/9 -> L4_Controller/9  "<FrontAxleLeftWheelSpeed>"
  Bus Selector/10 -> L4_Controller/10  "<FrontAxleRightWheelSpeed>"
  Bus Selector/11 -> L4_Controller/11  "<EBSBrakeSwitch>"
  Bus Selector/12 -> L4_Controller/12  "<SPN524_TransSelectedGear>"
  Bus Selector/13 -> L4_Controller/13  "<SPN523_TransCurrentGear>"
  Bus Selector/14 -> L4_Controller/14  "<SPN526_TransActualGearRatio>"
  Bus Selector/15 -> L4_Controller/15  "<ActualEngPercentTorque>"
  Bus Selector/16 -> L4_Controller/16  "<ActlEngPrcntTrqueHighResolution>"
  Bus Selector/17 -> L4_Controller/17  "<EngSpeed>"
  Bus Selector/18 -> L4_Controller/18  "<DriversDemandEngPercentTorque>"
  Bus Selector/19 -> L4_Controller/19  "<SPN514_NominalFrictionPercentTorque>"
  Bus Selector/20 -> L4_Controller/20  "<SPN2978_EstEngParasiticLossesPercentTorque>"
  Bus Selector/21 -> L4_Controller/21  "<SPN1760_GrossCombinationVehicleWeight>"
  Bus Selector/22 -> L4_Controller/22  "<ACCDistanceAlertSignal>"
  Bus Selector/23 -> L4_Controller/23  "<ForwardCollisionWarning>"
  Bus Selector/24 -> L4_Controller/24  "<SPN544_EngineReferenceTorque>"
  Bus Selector/25 -> L4_Controller/25  "<ROPEngCtrlActive>"
  Bus Selector/26 -> L4_Controller/26  "<ROPBrakeCtrlActive>"
  Bus Selector/27 -> L4_Controller/27  "<YCEngCtrlActive>"
  Bus Selector/28 -> L4_Controller/28  "<YCBrakeCtrlActive>"
  Bus Selector/29 -> L4_Controller/29  "<SteerWheelAngle>"
  Bus Selector/30 -> L4_Controller/30  "<YawRate>"
  Bus Selector/31 -> L4_Controller/31  "<BarometricPress>"
  Bus Selector/32 -> L4_Controller/32  "<AmbientAirTemp>"
  Bus Selector/33 -> L4_Controller/33  "<F_Truck1571_VIN_Match>"
  Bus Selector/34 -> L4_Controller/34  "<PitchAngleExRange>"
  Bus Selector/35 -> L4_Controller/35  "<Latitude_>"
  Bus Selector/36 -> L4_Controller/36  "<Longitude_>"
  Bus Selector/37 -> L4_Controller/37  "<HDOP_>"
  Bus Selector/38 -> L4_Controller/38  "<PX2_LanePosEstPosition>"
  Bus Selector/39 -> L4_Controller/39  "<PX2_LanePosEstAngle>"
  Bus Selector/40 -> L4_Controller/40  "<PX2_LanePosEstNumPoints>"
  Bus Selector/41 -> L4_Controller/41  "<F_Truck166_VIN_Match>"
  Bus Selector/42 -> L4_Controller/42  "<SPN1810_LongitudinalAcceleration>"
  Bus Selector/43 -> L4_Controller/43  "<SteerWheelTurnCounter>"
  Bus Selector/44 -> L4_Controller/44  "<SteerWheelAngleSensorType>"
  Bus Selector/45 -> L4_Controller/45  "<LateralAcceleration>"
  Bus Selector/46 -> L4_Controller/46  "<PIC_Bus>"
  Bus Selector/47 -> L4_Controller/47  "<XPRControlMode>"
  Bus Selector/48 -> L4_Controller/48  "<XPRErrorState>"
  Bus Selector/49 -> L4_Controller/49  "<PressureP1>"
  Bus Selector/50 -> L4_Controller/50  "<PressureP4>"
  Bus Selector/51 -> L4_Controller/51  "<PressureP21>"
  Bus Selector/52 -> L4_Controller/52  "<PressureP22>"
  Bus Selector/53 -> L4_Controller/53  "<PressureP42>"
  Bus Selector/54 -> L4_Controller/54  "<IgnitionKeySwitch_voltage>"
  Bus Selector/55 -> L4_Controller/55  "<Park_brake_switch>"
  Bus Selector/56 -> L4_Controller/56  "<CruiseCtrlEnableSwitch>"
  Bus Selector/2 -> L4_Controller/2  "<EnableSw>"
  Bus Selector/3 -> L4_Controller/3  "<EngagePB>"
  Bus Selector/57 -> L4_Controller/57  "<PropB_REAX_2_ActualHandwheelPos>"
  Bus Selector/58 -> L4_Controller/58  "<PropB_REAX_2_EchoedStrWhlPos>"
  Bus Selector/4 -> L4_Controller/4  "<LogEventPB>"
  Bus Selector/5 -> L4_Controller/5  "<BrakeSW>"

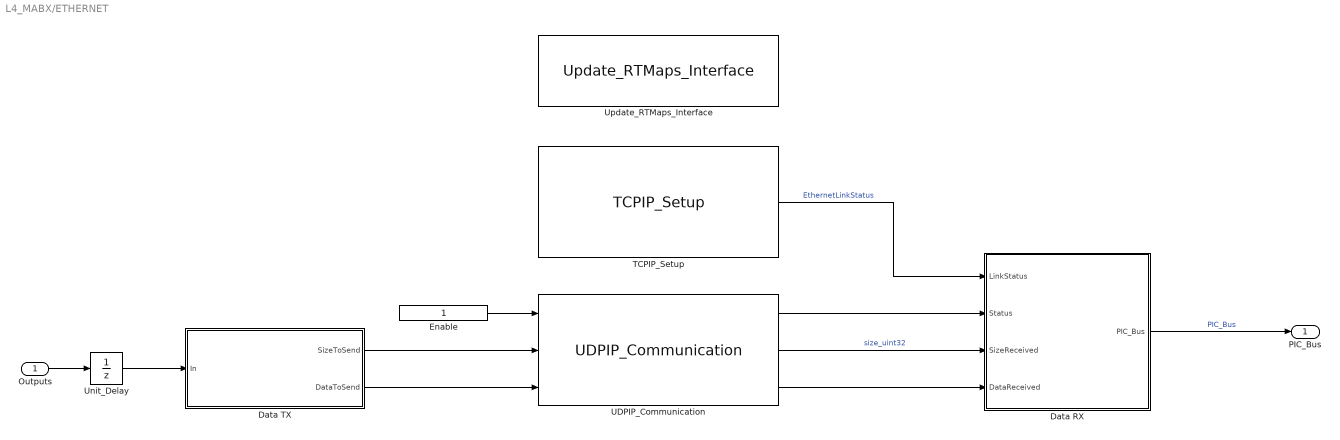
== system L4_MABX/ETHERNET ==
  Outputs : Inport
  Data RX : Subsystem
  Data TX : Subsystem
  Enable : Constant  OutDataTypeStr=boolean
  TCPIP_Setup : dsa_tcpip_lib/TCPIP_Setup  boardType=ETH Type 1  boardNo=1  channelNo=1  localIpAddr=10.120.128.20/23
      link override Interrupt_Task/Tcp Input Processing: TriggerPort=function-call  EnablePort=none  ThBlk=struct('blkh',92213.000122070313,'srcId','SWI1','srcSgnId','SWI1','intervalTmrBlockId',[],'srcSgnName',['Software Trigger'],'srcCpuId','','isSrcCpu',1,'isTargetCpu',1,'srcOnMasterCpu',1,'boardType','','boardTypeNo','','boardNo',1,'intNo',0,'subIntNo',-1,'period',0,'entryPoint','rti_SWI1','blockName',['Tcp Input Processing'],'taskNameDisplayExt','','taskType','SWINT','groupId','SWINT','hookFcn','NULL','isTimerTaskSrc',0,'service','','mpBlkId','','taskPriorityPreConfig','none','taskPriority',-1,'taskSortWeighting',[],'taskSchedulingPolicy','FCFS','taskOvrPreConfig','none','taskOvrStrategy',1,'taskOvrQueueSize',1,'taskVisibility','on','taskGroupId','','taskGroupDisplayOrder',[],'serviceDynamicGen',0,'disableCodeGen',0,'boardBase','0','noBoardBase','')  TLCFileName=rti_swinterrupt
      settings: SourceProductName=dSPACE MABX TCP/IP Blockset
  UDPIP_Communication : dsa_tcpip_lib/UDPIP_Communication  localPort=50000  remoteAddrStr=10.120.128.10  remotePort=50000  inputSize=24  outputSize=128  legacyMode=off
      settings: SourceProductName=dSPACE MABX TCP/IP Blockset
  Unit_Delay : UnitDelay  SampleTime=-1
      settings: AttributesFormatString=IC: %<vinit>
  Update_RTMaps_Interface : rtmapslib/Update_RTMaps_Interface  SystemSampleTime=-1
      settings: SourceProductName=dSPACE RTMaps Interface Blockset
  PIC_Bus : Outport
  wires:
  UDPIP_Communication/2 -> Data RX/3(SizeReceived)  "size_uint32"
  Outputs/1 -> Unit_Delay/1
  Data TX/1(SizeToSend) -> UDPIP_Communication/2
  Data TX/2(DataToSend) -> UDPIP_Communication/3
  UDPIP_Communication/1 -> Data RX/2(Status)
  TCPIP_Setup/1 -> Data RX/1(LinkStatus)  "EthernetLinkStatus"
  Data RX/1(PIC_Bus) -> PIC_Bus/1  "PIC_Bus"
  Enable/1 -> UDPIP_Communication/1
  UDPIP_Communication/3 -> Data RX/4(DataReceived)
  Unit_Delay/1 -> Data TX/1(In)

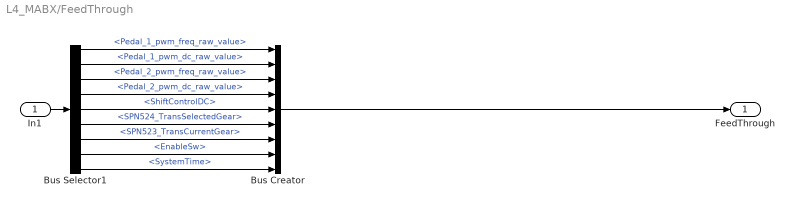
== system L4_MABX/FeedThrough ==
  In1 : Inport
  Bus Creator : BusCreator  Inputs=9
  Bus Selector1 : BusSelector  OutputSignals=DIO_Bus.Pedal_1_pwm_freq_raw_value,DIO_Bus.Pedal_1_pwm_dc_raw_value,DIO_Bus.Pedal_2_pwm_freq_raw_value,DIO_Bus.Pedal_2_pwm_dc_raw_value,DIO_Bus.ShiftControlDC,CAN.ETC2_03.SPN524_TransSelectedGear,CAN.ETC2_03.SPN523_TransCurrentGear,DIO_Bus.EnableSw,CAN.SystemTime
  FeedThrough : Outport
  wires:
  Bus Selector1/4 -> Bus Creator/4  "<Pedal_2_pwm_dc_raw_value>"
  Bus Selector1/2 -> Bus Creator/2  "<Pedal_1_pwm_dc_raw_value>"
  Bus Selector1/1 -> Bus Creator/1  "<Pedal_1_pwm_freq_raw_value>"
  Bus Selector1/3 -> Bus Creator/3  "<Pedal_2_pwm_freq_raw_value>"
  Bus Creator/1 -> FeedThrough/1
  Bus Selector1/7 -> Bus Creator/7  "<SPN523_TransCurrentGear>"
  Bus Selector1/9 -> Bus Creator/9  "<SystemTime>"
  Bus Selector1/5 -> Bus Creator/5  "<ShiftControlDC>"
  Bus Selector1/8 -> Bus Creator/8  "<EnableSw>"
  In1/1 -> Bus Selector1/1
  Bus Selector1/6 -> Bus Creator/6  "<SPN524_TransSelectedGear>"

== system L4_MABX/RTI Data ==
  RTI Data Store : Subsystem  Tag="struct('private',struct('version',struct('dsVer',uint32(2)),'access',struct('modified',['29-Jan-2020 16:07:02'],'type','Model','isPerm',1)),'public',struct('main',struct('data',[]),'sub',struct('name',{{'L4_MABX'}},'data',{{struct('TH',struct('thTaskInfo',struct('taskType',{'TIMER','HWINT','TMRINT','SWINT','GLINT'},'tasksNumOf',{9,1,1,1,0},'srcIds',{{'TIMERA','TIMERA2','TIMERA3','TIMERA4','TIMERA5','TIMERA6','TIMERA7','TIMERA8','TIMERA9'},{'BB_BYP_ETHT1M0I0S0'},{'TIMERB'},{'SWI1'},{}},'taskNames',{{['Timer Task 1'],['Timer Task 2'],['Timer Task 3'],['Timer Task 4'],['Timer Task 5'],['Timer Task 6'],['Timer Task 7'],['Timer Task 8'],['Timer Task 9']},{['MABXII_ETH_B1 HWINT0 Task']},{['Timer Interrupt']},{['Tcp Input Processing']},{}})),'th_tc',struct('dataType',{'TASK','TASK','TASK','TASK','TASK','TASK','TASK','TASK','TASK','TASK','TASK','TASK'},'taskGroupId',{'','','','','','','','','','','',''},'taskGroupList',{{},{},{},{},{},{},{},{},{},{},{},{}},'taskSchedulingPolicy',{'FCFS','FCFS','FCFS','FCFS','FCFS','FCFS','FCFS','FCFS','FCFS','FCFS','FCFS','FCFS'},'taskType',{'TIMER','TIMER','TIMER','TIMER','TIMER','TIMER','TIMER','TIMER','TIMER','HWINT','TMRINT','SWINT'},'blkh',{-1,-1,-1,-1,-1,-1,-1,-1,-1,['L4_MABX/ETHERNET/TCPIP_Setup/TCPIP_Interrupt_Block/Common Hardware' char(10) 'Interrupt Interface'],['L4_MABX/INPUTS_PIC_KW/Timer_Access/Timer Interrupt'],['L4_MABX/ETHERNET/TCPIP_Setup/Interrupt_Task/Tcp Input Processing']},'srcId',{'TIMERA','TIMERA2','TIMERA3','TIMERA4','TIMERA5','TIMERA6','TIMERA7','TIMERA8','TIMERA9','BB_BYP_ETHT1M0I0S0','TIMERB','SWI1'},'srcSgnName',{['Timer A interrupt'],['Timer Task 1'],['Timer Task 1'],['Timer Task 1'],['Timer Task 1'],['Timer Task 1'],['Timer Task 1'],['Timer Task 1'],['Timer Task 1'],['BB_BYP_ETH Type 1 Module 1 HW-Int 0 Interrupt 0'],['Timer B interrupt'],['Software Trigger']},'srcCpuName',{'','','','','','','','','','','',''},'taskName',{['Timer Task 1  [0.01] s'],['Timer Task 2  [0.02] s'],['Timer Task 3  [0.05] s'],['Timer Task 4  [0.1] s'],['Timer Task 5  [0.25] s'],['Timer Task 6  [0.5] s'],['Timer Task 7  [1] s'],['Timer Task 8  [5] s'],['Timer Task 9  [10] s'],['MABXII_ETH_B1 HWINT0 Task'],['Timer Interrupt'],['Tcp Input Processing']},'taskNameDisplayExt',{'','','','','','','','','','','',''},'smplTime',{0.01,0.02,0.05,0.1,2^-2,2^-1,1,5,10,0,0.01,0},'smplTimeOffs',{0,0,0,0,0,0,0,0,0,0,0,0},'hasFixedPriority',{0,0,0,0,0,0,0,0,0,0,0,0},'priority',{2,3,4,5,6,7,8,9,10,1,11,12},'hasFixedOvc',{0,0,0,0,0,0,0,0,0,0,0,0},'ovcType',{1,1,1,1,1,1,1,1,1,1,1,1},'ovcMax',{1,1,1,1,1,1,1,1,1,1,1,1}),'tc_th',struct('dataType',{'TASK','TASK','TASK','TASK','TASK','TASK','TASK','TASK','TASK','TASK','TASK','TASK'},'taskGroupId',{'','','','','','','','','','','',''},'taskGroupList',{{},{},{},{},{},{},{},{},{},{},{},{}},'taskSchedulingPolicy',{'FCFS','FCFS','FCFS','FCFS','FCFS','FCFS','FCFS','FCFS','FCFS','FCFS','FCFS','FCFS'},'taskType',{'TIMER','TIMER','TIMER','TIMER','TIMER','TIMER','TIMER','TIMER','TIMER','HWINT','TMRINT','SWINT'},'blkh',{-1,-1,-1,-1,-1,-1,-1,-1,-1,['L4_MABX/ETHERNET/TCPIP_Setup/TCPIP_Interrupt_Block/Common Hardware' char(10) 'Interrupt Interface'],['L4_MABX/INPUTS_PIC_KW/Timer_Access/Timer Interrupt'],['L4_MABX/ETHERNET/TCPIP_Setup/Interrupt_Task/Tcp Input Processing']},'srcId',{'TIMERA','TIMERA2','TIMERA3','TIMERA4','TIMERA5','TIMERA6','TIMERA7','TIMERA8','TIMERA9','BB_BYP_ETHT1M0I0S0','TIMERB','SWI1'},'srcSgnName',{['Timer A interrupt'],['Timer Task 1'],['Timer Task 1'],['Timer Task 1'],['Timer Task 1'],['Timer Task 1'],['Timer Task 1'],['Timer Task 1'],['Timer Task 1'],['BB_BYP_ETH Type 1 Module 1 HW-Int 0 Interrupt 0'],['Timer B interrupt'],['Software Trigger']},'srcCpuName',{'','','','','','','','','','','',''},'taskName',{['Timer Task 1  [0.01] s'],['Timer Task 2  [0.02] s'],['Timer Task 3  [0.05] s'],['Timer Task 4  [0.1] s'],['Timer Task 5  [0.25] s'],['Timer Task 6  [0.5] s'],['Timer Task 7  [1] s'],['Timer Task 8  [5] s'],['Timer Task 9  [10] s'],['MABXII_ETH_B1 HWINT0 Task'],['Timer Interrupt'],['Tcp Input Processing']},'taskNameDisplayExt',{'','','','','','','','','','','',''},'smplTime',{0.01,0.02,0.05,0.1,2^-2,2^-1,1,5,10,0,0.01,0},'smplTimeOffs',{0,0,0,0,0,0,0,0,0,0,0,0},'hasFixedPriority',{0,0,0,0,0,0,0,0,0,0,0,0},'priority',{2,3,4,5,6,7,8,9,10,1,11,12},'hasFixedOvc',{0,0,0,0,0,0,0,0,0,0,0,0},'ovcType',{1,1,1,1,1,1,1,1,1,1,1,1},'ovcMax',{1,1,1,1,1,1,1,1,1,1,1,1}))}})))"  mask(RTI_DATA_STORE){}
      mask help:
      | RTI Data Store Block. This block is used by RTI to store internal model dependent data. Deleting this block will result in data loss.
      |
      | NEVER DELETE, COPY, OR MODIFY THIS BLOCK!
      mask Help:
      | RTI Data Store Block. This block is used by RTI to store internal model dependent data. Deleting this block will result in data loss.
      | 
      | NEVER DELETE, COPY, OR MODIFY THIS BLOCK!
      mask Display: text(0.5, 0.5, ' ', 'HorizontalAlignment', 'center');

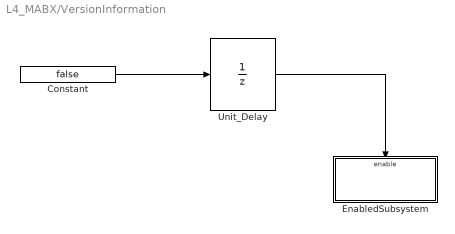
== system L4_MABX/VersionInformation ==
  Constant : Constant  Value=false
  EnabledSubsystem : Subsystem
  Unit_Delay : UnitDelay  InitialCondition=true  SampleTime=-1
      settings: AttributesFormatString=Init = %<InitialCondition>
  wires:
  Constant/1 -> Unit_Delay/1
  Unit_Delay/1 -> EnabledSubsystem/Enable
